simulink model "fel2"  (R2021a)
settings: Solver=VariableStepAuto  StartTime=0.0  StopTime=20  RelTol=1e-3
settings Model: Creator=Krisz  LastModifiedBy=Krisz

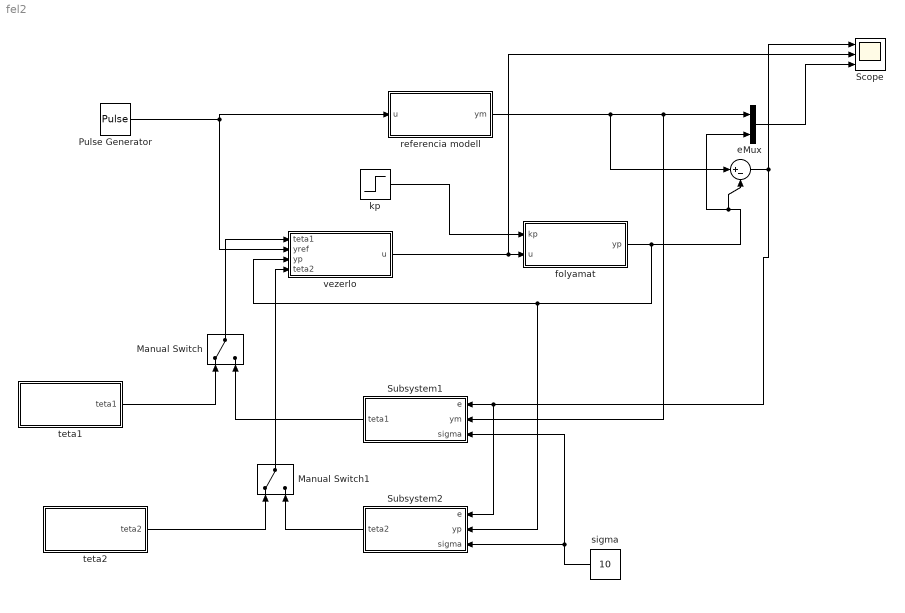
== system fel2 ==
  Manual Switch : ManualSwitch
  Manual Switch1 : ManualSwitch
  Mux : Mux  Inputs=2
  Pulse Generator : DiscretePulseGenerator  PulseType=Time based  Amplitude=5  Period=1  PulseWidth=50
  Scope : Scope  NumInputPorts=3
  Subsystem1 : Subsystem
  Subsystem2 : Subsystem
  e : Sum  Inputs=|+-
  folyamat : Subsystem
  kp : Step  Time=10  Before=2  After=8  SampleTime=0
  referencia modell : Subsystem
  sigma : Constant  Value=10
  teta1 : Subsystem
  teta2 : Subsystem
  vezerlo : Subsystem
  wires:
  Subsystem1/1(teta1) -> Manual Switch/2
  Pulse Generator/1 -> vezerlo/2(yref), referencia modell/1(u)
  referencia modell/1(ym) -> Mux/1, Subsystem1/2(ym), e/1
  e/1 -> Subsystem2/1(e), Subsystem1/1(e), Scope/1
  kp/1 -> folyamat/1(kp)
  teta1/1(teta1) -> Manual Switch/1
  Manual Switch/1 -> vezerlo/1(teta1)
  vezerlo/1(u) -> Scope/2, folyamat/2(u)
  folyamat/1(yp) -> Subsystem2/2(yp), vezerlo/3(yp), Mux/2, e/2
  Mux/1 -> Scope/3
  teta2/1(teta2) -> Manual Switch1/1
  Manual Switch1/1 -> vezerlo/4(teta2)
  sigma/1 -> Subsystem1/3(sigma), Subsystem2/3(sigma)
  Subsystem2/1(teta2) -> Manual Switch1/2

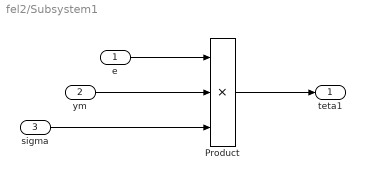
== system fel2/Subsystem1 ==
  e : Inport
  ym : Inport  Port=2
  sigma : Inport  Port=3
  Product : Product  Inputs=3
  teta1 : Outport
  wires:
  e/1 -> Product/1
  ym/1 -> Product/2
  Product/1 -> teta1/1
  sigma/1 -> Product/3

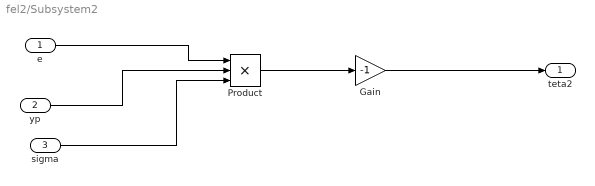
== system fel2/Subsystem2 ==
  e : Inport
  yp : Inport  Port=2
  sigma : Inport  Port=3
  Gain : Gain  Gain=-1
  Product : Product  Inputs=3
  teta2 : Outport
  wires:
  e/1 -> Product/1
  yp/1 -> Product/2
  sigma/1 -> Product/3
  Product/1 -> Gain/1
  Gain/1 -> teta2/1

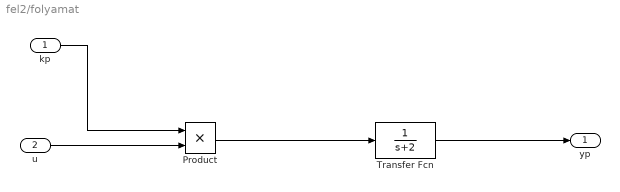
== system fel2/folyamat ==
  kp : Inport
  u : Inport  Port=2
  Product : Product
  Transfer Fcn : TransferFcn  Denominator=[1 2]
  yp : Outport
  wires:
  Product/1 -> Transfer Fcn/1
  Transfer Fcn/1 -> yp/1
  kp/1 -> Product/1
  u/1 -> Product/2

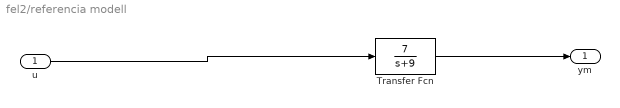
== system fel2/referencia modell ==
  u : Inport
  Transfer Fcn : TransferFcn  Numerator=[7]  Denominator=[1 9]
  ym : Outport
  wires:
  u/1 -> Transfer Fcn/1
  Transfer Fcn/1 -> ym/1

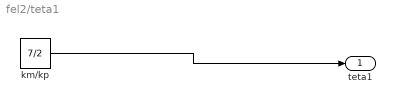
== system fel2/teta1 ==
  km/kp : Constant  Value=7/2
  teta1 : Outport
  wires:
  km/kp/1 -> teta1/1

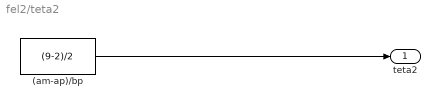
== system fel2/teta2 ==
  (am-ap)/bp : Constant  Value=(9-2)/2
  teta2 : Outport
  wires:
  (am-ap)/bp/1 -> teta2/1

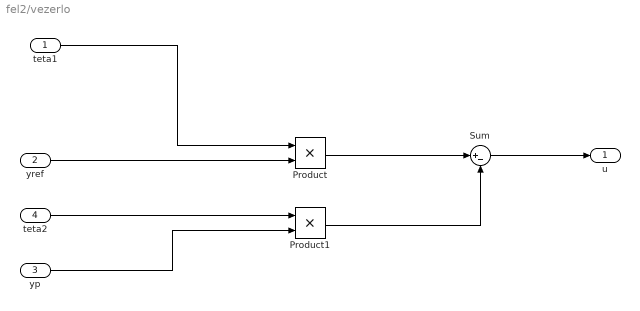
== system fel2/vezerlo ==
  teta1 : Inport
  yref : Inport  Port=2
  yp : Inport  Port=3
  teta2 : Inport  Port=4
  Product : Product
  Product1 : Product
  Sum : Sum  Inputs=|+-
  u : Outport
  wires:
  teta1/1 -> Product/1
  yref/1 -> Product/2
  teta2/1 -> Product1/1
  yp/1 -> Product1/2
  Product1/1 -> Sum/2
  Product/1 -> Sum/1
  Sum/1 -> u/1
